simulink model "puma560"  (R2015a)
settings: Solver=ode45  StartTime=0.0  StopTime=inf  RelTol=1e-3
libraries: robotlib x10
settings Model: Creator=jwcjdenissen  LastModifiedBy=jwcjdenissen
settings DebuggingCC: UnconnectedInputMsg=none  UnconnectedOutputMsg=none  UnconnectedLineMsg=none

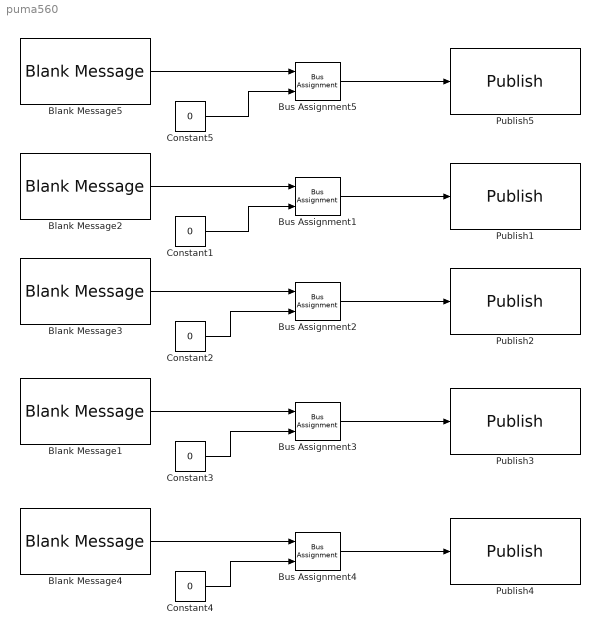
== system puma560 ==
  Blank Message{1..5} (5 alike) : robotlib/Blank Message  SourceLibraryInfo=This block requires Robotics System Toolbox  messageType=std_msgs/Float64  SampleTime=inf
  Bus Assignment{1..5} (5 alike) : BusAssignment  AssignedSignals=Data
  Constant{1..5} (5 alike) : Constant  Value=0
  Publish1 : robotlib/Publish  SourceLibraryInfo=This block requires Robotics System Toolbox  topicSource=Specify your own  topic=/puma560/joint_2_position_controller/command  messageType=std_msgs/Float64  messageQueueLength=1
  Publish2 : robotlib/Publish  SourceLibraryInfo=This block requires Robotics System Toolbox  topicSource=Specify your own  topic=/puma560/joint_3_position_controller/command  messageType=std_msgs/Float64  messageQueueLength=1
  Publish3 : robotlib/Publish  SourceLibraryInfo=This block requires Robotics System Toolbox  topicSource=Specify your own  topic=/puma560/joint_4_position_controller/command  messageType=std_msgs/Float64  messageQueueLength=1
  Publish4 : robotlib/Publish  SourceLibraryInfo=This block requires Robotics System Toolbox  topicSource=Specify your own  topic=/puma560/joint_5_position_controller/command  messageType=std_msgs/Float64  messageQueueLength=1
  Publish5 : robotlib/Publish  SourceLibraryInfo=This block requires Robotics System Toolbox  topicSource=Specify your own  topic=/puma560/joint_1_position_controller/command  messageType=std_msgs/Float64  messageQueueLength=1
  wires:
  Bus Assignment1/1 -> Publish1/1
  Blank Message2/1 -> Bus Assignment1/1
  Bus Assignment2/1 -> Publish2/1
  Blank Message3/1 -> Bus Assignment2/1
  Constant2/1 -> Bus Assignment2/2
  Bus Assignment3/1 -> Publish3/1
  Blank Message1/1 -> Bus Assignment3/1
  Constant3/1 -> Bus Assignment3/2
  Bus Assignment4/1 -> Publish4/1
  Blank Message4/1 -> Bus Assignment4/1
  Constant4/1 -> Bus Assignment4/2
  Constant1/1 -> Bus Assignment1/2
  Bus Assignment5/1 -> Publish5/1
  Blank Message5/1 -> Bus Assignment5/1
  Constant5/1 -> Bus Assignment5/2
